simulink model "PCH_660_400_x3_6arm"  (R2018b)
settings: Solver=ode23t  StartTime=0.0  StopTime=0.1  RelTol=1e-3
undefined symbols (not defined in the file): fn, L_load, Lk, R12pu, R_load, Rmpu, Stv, U1, U2, X12pu, Xmpu
libraries: powerlib x65, powerlib_meascontrol x20, peRmsMeasurement x4
settings Model: Creator=K2  LastModifiedBy=sr1

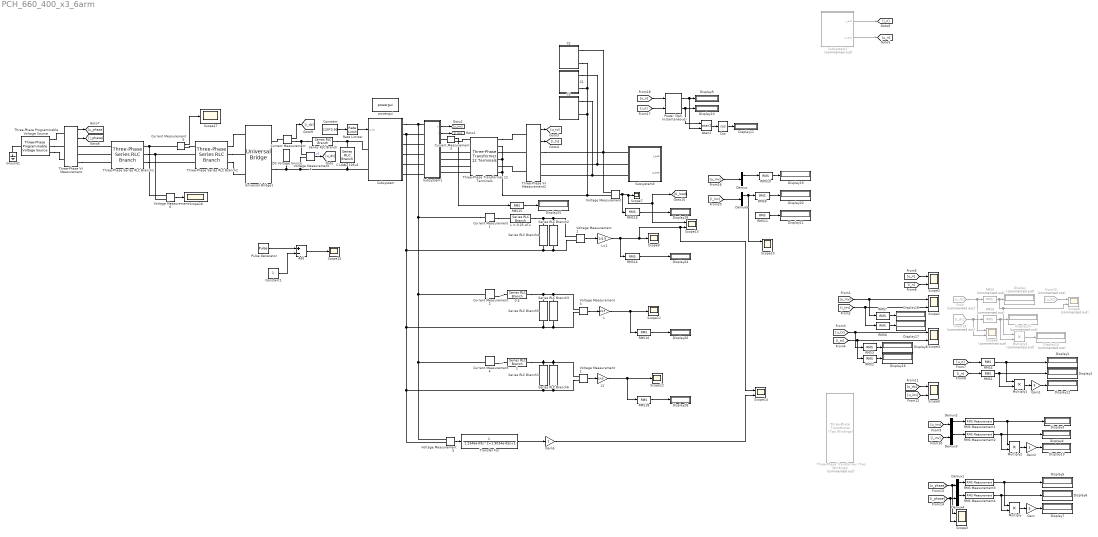
== system PCH_660_400_x3_6arm ==
  0.5 : powerlib/Elements/Series RLC Branch  LConnTagsString=__new0  RConnTagsString=__new0  BranchType=L  Resistance=0.0001  Inductance=Lk*2  SetiL0=off  InitialCurrent=0  Capacitance=1e-6  Setx0=off  InitialVoltage=0  Measurements=None
  1 : powerlib/Elements/Series RLC Branch  LConnTagsString=__new0  RConnTagsString=__new0  BranchType=L  Resistance=0.0001  Inductance=Lk*4  SetiL0=off  InitialCurrent=0  Capacitance=1e-6  Setx0=off  InitialVoltage=0  Measurements=None
  Add : Sum  Inputs=+-
  Atan2 : Trigonometry  Operator=atan2
  C1 : Subsystem
  C2 : Subsystem
  C3 : Subsystem
  Constant : Constant  Value=120*0.90  SampleTime=1e-6
  Constant1 : Constant
  Cos : Trigonometry  Operator=cos
  Current Measurement{,1..5} (6 alike) : powerlib/Measurements/Current Measurement  PhasorSimulation=off  OutputType=Complex  PSBequivalent=0
  DC Voltage Source : powerlib/Electrical Sources/DC Voltage Source  Amplitude=510*0.9  Measurements=None
  Demux{,1..5} (6 alike) : Demux  Outputs=3
  Display : Display  Commented=on
  Display{1..13,16..21,24..26,28..29} (24 alike) : Display
  Display14 : Display  Commented=on
  Display15 : Display  Commented=on
  From : From  Commented=on  GotoTag=u_dc
  From15 : From  Commented=on  GotoTag=u_dc
  From19 : From  Commented=on  GotoTag=i_dc
  Gain : Gain  Gain=3
  Gain1 : Gain  Gain=3
  Gain2 : Gain  Gain=3
  Gain5 : Gain
  Ground1 : powerlib/Elements/Ground  LConnTagsString=a
  L : Gain  Gain=1/4.5
  L = 0.25 мГн : powerlib/Elements/Series RLC Branch  LConnTagsString=__new0  RConnTagsString=__new0  BranchType=L  Resistance=0.002  Inductance=Lk  SetiL0=off  InitialCurrent=0  Capacitance=1e-6  Setx0=off  InitialVoltage=0  Measurements=None
  L1 : Gain  Gain=1/4.5
  "L=1 " : Gain  Gain=1/4.5
  Multiply : Product
  Multiply1 : Product
  Multiply2 : Product
  Multiply3 : Product  Commented=on
  "Power (3ph, Instantaneous)" : powerlib_meascontrol/Measurements/Power (3ph, Instantaneous)
      settings: SourceProductName=Simscape Power Systems
  Pulse Generator : DiscretePulseGenerator  PulseType=Time based  Amplitude=2  Period=1/400  PulseWidth=50
  RMS Measurement1 : peRmsMeasurement/RMS Measurement  LabelModeActiveChoice=Harmonic  F=400  SpecifyHarmonics=on  K=[1]  Ts=0
  RMS Measurement2 : peRmsMeasurement/RMS Measurement  LabelModeActiveChoice=Harmonic  F=400  SpecifyHarmonics=on  K=[1]  Ts=0
  RMS Measurement3 : peRmsMeasurement/RMS Measurement  LabelModeActiveChoice=Harmonic  F=50  SpecifyHarmonics=on  K=[1]  Ts=0
  RMS Measurement4 : peRmsMeasurement/RMS Measurement  LabelModeActiveChoice=Harmonic  F=50  SpecifyHarmonics=on  K=[1]  Ts=0
  RMS{1..4,6..7,9..11,14..16,18..19} (14 alike) : powerlib_meascontrol/Measurements/RMS  TrueRMS=on  Freq=400  RMSInit=0  Ts=0
  RMS5 : powerlib_meascontrol/Measurements/RMS  Commented=on  TrueRMS=on  Freq=300  RMSInit=0  Ts=0
  RMS8 : powerlib_meascontrol/Measurements/RMS  Commented=on  TrueRMS=on  Freq=300  RMSInit=0  Ts=0
  Rate Limiter : RateLimiter  RisingSlewLimit=50000  FallingSlewLimit=-50000  SampleTimeMode=inherited
  Scope{1..5,10,13..14} (8 alike) : Scope  NumInputPorts=2
  Scope{7,9,11..12,15..17} (7 alike) : Scope
  Scope6 : Scope  Commented=on  NumInputPorts=2
  Scope8 : Scope  Commented=on  NumInputPorts=2
  Series RLC Branch : powerlib/Elements/Series RLC Branch  LConnTagsString=__new0  RConnTagsString=__new0  BranchType=R  Resistance=0.0001  Inductance=250e-6  SetiL0=off  InitialCurrent=0  Capacitance=1e-6  Setx0=off  InitialVoltage=0  Measurements=None
  Series RLC Branch1 : powerlib/Elements/Series RLC Branch  LConnTagsString=__new0  RConnTagsString=__new0  BranchType=C  Resistance=0.0001  Inductance=250e-6  SetiL0=off  InitialCurrent=0  Capacitance=100e-6 / ((4.5)^2)  Setx0=off  InitialVoltage=0  Measurements=None
  Series RLC Branch2 : powerlib/Elements/Series RLC Branch  LConnTagsString=__new0  RConnTagsString=__new0  BranchType=R  Resistance=R_load * ((4.5)^2)  Inductance=250e-6  SetiL0=off  InitialCurrent=0  Capacitance=100e-6 / ((4.5)^2)  Setx0=off  InitialVoltage=0  Measurements=None
  Series RLC Branch3 : powerlib/Elements/Series RLC Branch  LConnTagsString=__new0  RConnTagsString=__new0  BranchType=R  Resistance=R_load * ((4.5)^2)  Inductance=250e-6  SetiL0=off  InitialCurrent=0  Capacitance=100e-6 / ((4.5)^2)  Setx0=off  InitialVoltage=0  Measurements=None
  Series RLC Branch4 : powerlib/Elements/Series RLC Branch  LConnTagsString=__new0  RConnTagsString=__new0  BranchType=C  Resistance=0.0001  Inductance=250e-6  SetiL0=off  InitialCurrent=0  Capacitance=100e-6 / ((4.5)^2)  Setx0=off  InitialVoltage=0  Measurements=None
  Series RLC Branch5 : powerlib/Elements/Series RLC Branch  LConnTagsString=__new0  RConnTagsString=__new0  BranchType=C  Resistance=0.0001  Inductance=250e-6  SetiL0=off  InitialCurrent=0  Capacitance=100e-6 / ((4.5)^2)  Setx0=off  InitialVoltage=0  Measurements=None
  Series RLC Branch6 : powerlib/Elements/Series RLC Branch  LConnTagsString=__new0  RConnTagsString=__new0  BranchType=R  Resistance=R_load * ((4.5)^2)  Inductance=250e-6  SetiL0=off  InitialCurrent=0  Capacitance=100e-6 / ((4.5)^2)  Setx0=off  InitialVoltage=0  Measurements=None
  Subsystem : Subsystem
  Subsystem1 : Subsystem
  Subsystem2 : Subsystem  Commented=on
  Subsystem3 : Subsystem
  Three-Phase Programmable Voltage Source : powerlib/Electrical Sources/Three-Phase Programmable Voltage Source  PositiveSequence=[660 0 50]  VariationEntity=None  VariationType=Table of time-amplitude pairs  VariationTypeAlt=Step  VariationStep=0.5  VariationRate=10  VariationMagnitude=0.3  VariationFrequency=2  VariationTiming=[1 2]  VariationPhaseA=off  Amplitudes=[1 0.8 1.2 1.0]  TimeValues=[0 0.1 0.15 0.2]  HarmonicGeneration=off  HarmonicA=[3 0.2 -25 0]  HarmonicB=[2 0.15 35 2]  Timing="[0.05  3]"  BusType=swing  Pref=0  Qref=0  Qmin=-inf  Qmax=inf
  Three-Phase Series RLC Branch1 : powerlib/Elements/Three-Phase Series RLC Branch  LConnTagsString=A|B|C  RConnTagsString=A|B|C  BranchType=R  Resistance=0.18  Inductance=150e-6  Capacitance=1e-6  Measurements=None
  Three-Phase Series RLC Branch2 : powerlib/Elements/Three-Phase Series RLC Branch  LConnTagsString=A|B|C  RConnTagsString=A|B|C  BranchType=L  Resistance=1  Inductance=150e-6  Capacitance=1e-6  Measurements=None
  Three-Phase Transformer (Two Windings) : powerlib/Elements/Three-Phase Transformer (Two Windings)  Commented=on  Winding1Connection=Yg  Winding2Connection=Yg  CoreType=Three single-phase transformers  SetSaturation=off  Hysteresis=off  DataFile='hysteresis'  SetInitialFlux=off  Measurements=None  UNITS=pu  NominalPower=[ 160e3 , 400 ]  Winding1=[690 , 0.002 , 0.08 ]  Winding2=[ 230 , 0.002 , 0.08 ]  Rm=500  Lm=500  L0=0.5  Saturation=[ 0,0 ; 0.0024,1.2 ; 1.0,1.52 ]  InitialFluxes=[ 0.8 , -0.8 , 0.7 ]  MoreParameters=off  BreakLoop=off  DataType=off  TransfoNumber=1
  Three-Phase V-I Measurement : powerlib/Measurements/Three-Phase V-I Measurement  VoltageMeasurement=phase-to-ground  SetLabelV=off  LabelV=Vabc  Vpu=off  VpuLL=off  CurrentMeasurement=yes  SetLabelI=off  LabelI=Iabc  Ipu=off  Pbase=100e6  Vbase=500e3  OutputType=Complex  PhasorSimulation=off  PSBequivalent=0
  Three-Phase V-I Measurement2 : powerlib/Measurements/Three-Phase V-I Measurement  VoltageMeasurement=phase-to-phase  SetLabelV=off  LabelV=Vabc  Vpu=off  VpuLL=off  CurrentMeasurement=yes  SetLabelI=off  LabelI=Iabc  Ipu=off  Pbase=100e6  Vbase=500e3  OutputType=Complex  PhasorSimulation=off  PSBequivalent=0
  Three-Phase Transformer 12 Terminals : powerlib/Elements/Three-Phase Transformer 12 Terminals  RatedPower=[ Stv fn ]  Winding1="[ U1 R12pu  X12pu ]"  Winding2=[ U2 R12pu X12pu]  RmXm=[ Rmpu Xmpu ]
      settings: SourceProductName=Simscape Power Systems  SourceProductBaseCode=PS
  Transfer Fcn : TransferFcn  Denominator=[1.2346e-09 1.9034e-05 1]
  Universal Bridge1 : powerlib/Power Electronics/Universal Bridge  Arms=3  SnubberResistance=1e5  SnubberCapacitance=inf  Device=Diodes  Ron=1e-3  Lon=0  ForwardVoltages="[  0  0  ]"  ForwardVoltage=0  GTOparameters=[ 10e-6 , 20e-6 ]  IGBTparameters=[ 1e-6 , 2e-6 ]  Measurements=None  Measurements_2=None  converterType=Rectifier
  Voltage Measurement{,1..6} (7 alike) : powerlib/Measurements/Voltage Measurement  PhasorSimulation=off  OutputType=Complex  PSBequivalent=0
  powergui : powerlib/powergui  Priority=1  SimulationMode=Discrete  SampleTime=1e-6  frequency=60  Iterations=50  frequencyindice=0  Pbase=100e6  ErrMax=1e-4  UnitsV=kV  UnitsW=MW  buscounter=0  FunctionMessages=off  echomessages=off  EnableUseOfTLC=off  CurrentSourceSwitches=off  DisableSnubberDevices=off  DisableRonSwitches=off  DisableVfSwitches=off  DisplayEquations=off  SolverType=Tustin/Backward Euler (TBE)  Interpol=off  ExternalGateDelay=off  methode=off  Ts=100  x0status=blocks  SPID=on  SwTol=0  HookPort=off  RestoreLinks=warning  ResistiveCurrentMeasurement=off  Frange=[0:2:500]  Ylog=off  Xlog=on  ShowGrid=off  save=off  variable=ZData  structure=logsout  ZoomFFT=off  StartTime=0.08  cycles=4  DisplayStyle=1  fundamental=400  FreqAxis=off  MaxFrequency=4000  frequencyindicesteady=1  RmsSteady=1  display=off
  С LOAD 105u1 : powerlib/Elements/Series RLC Branch  LConnTagsString=__new0  RConnTagsString=__new0  BranchType=C  Resistance=250*250/50e3  Inductance=1e-3  SetiL0=off  InitialCurrent=0  Capacitance=11400e-6  Setx0=on  InitialVoltage=800  Measurements=None
  wires:
  Three-Phase V-I Measurement/1 -> [u_phase]
  Three-Phase V-I Measurement/2 -> [i_phase]
  Voltage Measurement4/1 -> [u_dc]  "u1"
  Three-Phase V-I Measurement2/1 -> [u_tv]
  Three-Phase V-I Measurement2/2 -> [i_tv]
  Constant/1 -> Rate Limiter/1
  [u_n] -> Scope2/1
  [i_n] -> Scope2/2
  [u_inv] -> RMS7/1, Scope1/1
  [i_inv] -> RMS6/1, Scope1/2
  [u_tv] -> Scope4/1, RMS3/1
  [i_tv] -> Scope4/2, RMS2/1
  [u_n] -> RMS4/1
  [i_n] -> RMS1/1
  [i_inv] -> Demux3/1
  [u_inv] -> Demux2/1
  [u_dc] -> Scope5/1
  [u_inv] -> Scope5/2
  Rate Limiter/1 -> Subsystem/1(u in)
  RMS5/1 -> Multiply3/1, Scope6/2, Display/1
  RMS Measurement3/1 -> Multiply/1, Display5/1
  RMS Measurement4/1 -> Multiply/2, Display6/1
  Multiply/1 -> Gain/1
  Gain/1 -> Display7/1
  From15/1 -> Scope6/1
  Subsystem1/2(i) -> [i_inv]
  Subsystem1/1(v) -> [u_inv]
  Cos/1 -> Display11/1
  "Power (3ph, Instantaneous)"/2 -> Atan2/1, Display10/1
  Atan2/1 -> Cos/1
  "Power (3ph, Instantaneous)"/1 -> Atan2/2, Display9/1
  [i_n] -> "Power (3ph, Instantaneous)"/2
  [u_n] -> "Power (3ph, Instantaneous)"/1
  Gain1/1 -> Display12/1
  RMS1/1 -> Display2/1, Multiply1/2
  RMS4/1 -> Display1/1, Multiply1/1
  Multiply1/1 -> Gain1/1
  Gain2/1 -> Display13/1
  RMS Measurement2/1 -> Multiply2/2, Display4/1
  RMS Measurement1/1 -> Multiply2/1, Display3/1
  Multiply2/1 -> Gain2/1
  Current Measurement/1 -> [i_dc]
  RMS8/1 -> Multiply3/2, Display14/1
  Multiply3/1 -> Display15/1
  From/1 -> Scope8/1, RMS5/1
  From19/1 -> Scope8/2, RMS8/1
  Demux2/1 -> RMS Measurement1/1
  Demux3/1 -> RMS Measurement2/1
  Demux4/1 -> RMS Measurement4/1
  Demux1/1 -> RMS Measurement3/1
  [u_phase] -> Scope3/1, Demux1/1
  [i_phase] -> Scope3/2, Demux4/1
  RMS3/1 -> Display8/1
  RMS2/1 -> Display16/1
  RMS6/1 -> Display17/1
  RMS7/1 -> Display18/1
  Voltage Measurement1/1 -> "L=1 "/1
  Voltage Measurement3/1 -> L/1
  Voltage Measurement5/1 -> Transfer Fcn/1
  Transfer Fcn/1 -> Gain5/1
  "L=1 "/1 -> RMS14/1, Scope14/1, Scope13/2, Scope9/1
  RMS10/1 -> Display19/1
  [u_inv] -> Demux/1
  Demux/1 -> RMS10/1
  RMS9/1 -> Display20/1
  RMS11/1 -> Display21/1
  Demux5/1 -> Scope10/1, RMS9/1
  [i_inv] -> Demux5/1
  Subsystem2/1(i_out) -> [i_n]
  Subsystem2/2(u_out) -> [u_n]
  RMS14/1 -> Display24/1
  RMS16/1 -> Display26/1
  RMS15/1 -> Display25/1
  Current Measurement3/1 -> RMS15/1
  Voltage Measurement2/1 -> L1/1
  L1/1 -> RMS18/1, Scope12/1
  RMS18/1 -> Display28/1
  RMS19/1 -> Display29/1
  Voltage Measurement/1 -> [U_load], Scope13/1, Scope7/1, RMS19/1
  Gain5/1 -> Scope14/2
  L/1 -> RMS16/1, Scope11/1
  Pulse Generator/1 -> Add/1
  Constant1/1 -> Add/2
  Add/1 -> Scope15/1
  Voltage Measurement6/1 -> Scope16/1
  Current Measurement5/1 -> Scope17/1
  connections:
  Three-Phase Programmable Voltage Source/RConn3 -- Three-Phase V-I Measurement/LConn3
  Three-Phase Programmable Voltage Source/RConn2 -- Three-Phase V-I Measurement/LConn2
  Three-Phase Series RLC Branch2/RConn3 -- Universal Bridge1/LConn3
  Three-Phase Programmable Voltage Source/LConn1 -- Ground1/LConn1
  Three-Phase Series RLC Branch2/RConn1 -- Universal Bridge1/LConn1
  Three-Phase Programmable Voltage Source/RConn1 -- Three-Phase V-I Measurement/LConn1
  Three-Phase Series RLC Branch2/RConn2 -- Universal Bridge1/LConn2
  Series RLC Branch/LConn1 -- Current Measurement/RConn1 -- Voltage Measurement4/LConn1
  Universal Bridge1/RConn2 -- Subsystem/LConn2 -- С LOAD 105u1/RConn1 -- Voltage Measurement4/LConn2 -- DC Voltage Source/LConn1
  Three-Phase V-I Measurement2/RConn1 -- Subsystem3/LConn1 -- Voltage Measurement/LConn1 -- C2/LConn1
  C3/LConn1 -- Three-Phase V-I Measurement2/RConn3 -- Subsystem3/LConn3
  Three-Phase V-I Measurement2/LConn2 -- Three-Phase Transformer 12 Terminals/RConn3
  Three-Phase Transformer 12 Terminals/RConn1 -- Three-Phase V-I Measurement2/LConn1
  Series RLC Branch/RConn1 -- Subsystem/LConn1 -- С LOAD 105u1/LConn1
  Voltage Measurement2/LConn2 -- Series RLC Branch5/RConn1 -- Series RLC Branch3/RConn1 -- Voltage Measurement3/LConn2 -- Series RLC Branch2/RConn1 -- Voltage Measurement1/LConn2 -- Series RLC Branch4/RConn1 -- Subsystem/RConn2 -- Subsystem1/LConn2 -- Voltage Measurement5/LConn2 -- Series RLC Branch1/RConn1 -- Series RLC Branch6/RConn1
  Three-Phase Transformer 12 Terminals/LConn4 -- Subsystem1/RConn4
  Three-Phase Transformer 12 Terminals/LConn5 -- Subsystem1/RConn5
  Three-Phase Transformer 12 Terminals/LConn3 -- Subsystem1/RConn3
  Current Measurement1/LConn1 -- Voltage Measurement5/LConn1 -- Current Measurement4/LConn1 -- Current Measurement2/LConn1 -- Subsystem/RConn1 -- Subsystem1/LConn1
  Subsystem1/LConn3 -- Subsystem/RConn3
  Subsystem1/LConn4 -- Subsystem/RConn4
  Subsystem1/LConn5 -- Subsystem/RConn5
  Subsystem1/LConn6 -- Subsystem/RConn6
  Current Measurement/LConn1 -- Universal Bridge1/RConn1
  Three-Phase V-I Measurement2/LConn3 -- Three-Phase Transformer 12 Terminals/RConn5
  C1/LConn1 -- Three-Phase V-I Measurement2/RConn2 -- Subsystem3/LConn2
  C2/LConn3 -- C1/LConn3 -- C3/LConn3 -- Voltage Measurement/LConn2 -- Three-Phase Transformer 12 Terminals/RConn2 -- Three-Phase Transformer 12 Terminals/RConn4 -- Three-Phase Transformer 12 Terminals/RConn6
  L = 0.25 мГн/RConn1 -- Series RLC Branch2/LConn1 -- Voltage Measurement1/LConn1 -- Series RLC Branch4/LConn1
  Current Measurement1/RConn1 -- L = 0.25 мГн/LConn1
  Three-Phase Transformer 12 Terminals/LConn2 -- Subsystem1/RConn2
  Three-Phase Transformer 12 Terminals/LConn6 -- Subsystem1/RConn6
  Current Measurement2/RConn1 -- 0.5/LConn1
  Current Measurement3/RConn1 -- Three-Phase Transformer 12 Terminals/LConn1
  Current Measurement3/LConn1 -- Subsystem1/RConn1
  Series RLC Branch1/LConn1 -- Series RLC Branch6/LConn1 -- Voltage Measurement2/LConn1 -- 1/RConn1
  Current Measurement4/RConn1 -- 1/LConn1
  0.5/RConn1 -- Series RLC Branch3/LConn1 -- Voltage Measurement3/LConn1 -- Series RLC Branch5/LConn1
  Three-Phase Series RLC Branch1/RConn1 -- Current Measurement5/LConn1 -- Voltage Measurement6/LConn1
  Three-Phase Series RLC Branch1/LConn1 -- Three-Phase V-I Measurement/RConn1
  Three-Phase Series RLC Branch1/RConn2 -- Three-Phase Series RLC Branch2/LConn2 -- Voltage Measurement6/LConn2
  Three-Phase Series RLC Branch1/LConn2 -- Three-Phase V-I Measurement/RConn2
  Three-Phase V-I Measurement/RConn3 -- Three-Phase Series RLC Branch1/LConn3
  Three-Phase Series RLC Branch1/RConn3 -- Three-Phase Series RLC Branch2/LConn3
  Current Measurement5/RConn1 -- Three-Phase Series RLC Branch2/LConn1

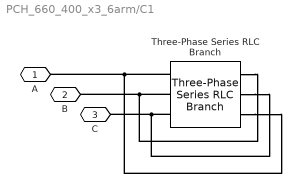
== system PCH_660_400_x3_6arm/C1 ==
  Three-Phase Series RLC Branch : powerlib/Elements/Three-Phase Series RLC Branch  LConnTagsString=A|B|C  RConnTagsString=A|B|C  BranchType=C  Resistance=0.001  Inductance=100e-6  Capacitance=100e-6  Measurements=None
  A : PMIOPort  Side=Left
  B : PMIOPort  Port=2  Side=Left
  C : PMIOPort  Port=3  Side=Left
  connections:
  Three-Phase Series RLC Branch/LConn3 -- Three-Phase Series RLC Branch/RConn2 -- C/RConn1
  Three-Phase Series RLC Branch/LConn1 -- Three-Phase Series RLC Branch/RConn3 -- A/RConn1
  Three-Phase Series RLC Branch/LConn2 -- Three-Phase Series RLC Branch/RConn1 -- B/RConn1

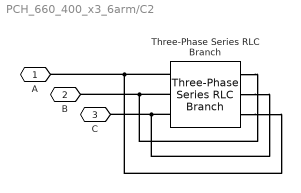
== system PCH_660_400_x3_6arm/C2 ==
  Three-Phase Series RLC Branch : powerlib/Elements/Three-Phase Series RLC Branch  LConnTagsString=A|B|C  RConnTagsString=A|B|C  BranchType=C  Resistance=0.001  Inductance=100e-6  Capacitance=100e-6  Measurements=None
  A : PMIOPort  Side=Left
  B : PMIOPort  Port=2  Side=Left
  C : PMIOPort  Port=3  Side=Left
  connections:
  Three-Phase Series RLC Branch/LConn3 -- Three-Phase Series RLC Branch/RConn2 -- C/RConn1
  Three-Phase Series RLC Branch/LConn1 -- Three-Phase Series RLC Branch/RConn3 -- A/RConn1
  Three-Phase Series RLC Branch/LConn2 -- Three-Phase Series RLC Branch/RConn1 -- B/RConn1

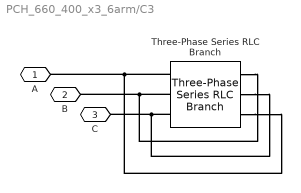
== system PCH_660_400_x3_6arm/C3 ==
  Three-Phase Series RLC Branch : powerlib/Elements/Three-Phase Series RLC Branch  LConnTagsString=A|B|C  RConnTagsString=A|B|C  BranchType=C  Resistance=0.001  Inductance=100e-6  Capacitance=100e-6  Measurements=None
  A : PMIOPort  Side=Left
  B : PMIOPort  Port=2  Side=Left
  C : PMIOPort  Port=3  Side=Left
  connections:
  Three-Phase Series RLC Branch/LConn3 -- Three-Phase Series RLC Branch/RConn2 -- C/RConn1
  Three-Phase Series RLC Branch/LConn1 -- Three-Phase Series RLC Branch/RConn3 -- A/RConn1
  Three-Phase Series RLC Branch/LConn2 -- Three-Phase Series RLC Branch/RConn1 -- B/RConn1

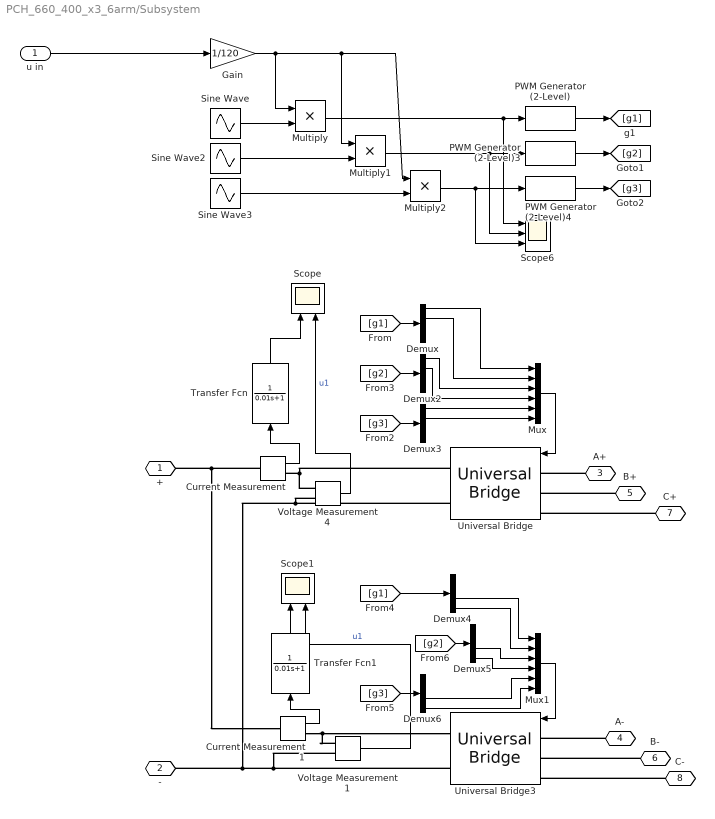
== system PCH_660_400_x3_6arm/Subsystem ==
  u in : Inport
  Current Measurement : powerlib/Measurements/Current Measurement  PhasorSimulation=off  OutputType=Complex  PSBequivalent=0
  Current Measurement1 : powerlib/Measurements/Current Measurement  PhasorSimulation=off  OutputType=Complex  PSBequivalent=0
  Demux{,2..6} (6 alike) : Demux
  Gain : Gain  Gain=1/120
  Multiply : Product
  Multiply1 : Product
  Multiply2 : Product
  Mux : Mux  Inputs=6
  Mux1 : Mux  Inputs=6
  PWM Generator (2-Level) : powerlib_meascontrol/Pulse & Signal Generators/PWM Generator (2-Level)  ModulatorType=Single-phase full-bridge (4 pulses)  ModulatorMode=Unsynchronized  Fc=5600  Pc=0  nF=27  MinMax="[ -1  1 ]"  SamplingTechnique=Natural  ModulatingSignals=off  m=0.8  Freq=60  Phase=0  Ts=0  ShowCarrierOutport=off
      settings: SourceProductName=Simscape Power Systems
  PWM Generator (2-Level)3 : powerlib_meascontrol/Pulse & Signal Generators/PWM Generator (2-Level)  ModulatorType=Single-phase full-bridge (4 pulses)  ModulatorMode=Unsynchronized  Fc=5600  Pc=120  nF=27  MinMax="[ -1  1 ]"  SamplingTechnique=Natural  ModulatingSignals=off  m=0.8  Freq=60  Phase=0  Ts=0  ShowCarrierOutport=off
      settings: SourceProductName=Simscape Power Systems
  PWM Generator (2-Level)4 : powerlib_meascontrol/Pulse & Signal Generators/PWM Generator (2-Level)  ModulatorType=Single-phase full-bridge (4 pulses)  ModulatorMode=Unsynchronized  Fc=5600  Pc=-120  nF=27  MinMax="[ -1  1 ]"  SamplingTechnique=Natural  ModulatingSignals=off  m=0.8  Freq=60  Phase=0  Ts=0  ShowCarrierOutport=off
      settings: SourceProductName=Simscape Power Systems
  Scope : Scope  NumInputPorts=2
  Scope1 : Scope  NumInputPorts=2
  Scope6 : Scope  NumInputPorts=3
  Sine Wave : Sin  Frequency=400*2*pi  SampleTime=0
  Sine Wave2 : Sin  Frequency=400*2*pi  Phase=-2*pi/3  SampleTime=0
  Sine Wave3 : Sin  Frequency=400*2*pi  Phase=2*pi/3  SampleTime=0
  Transfer Fcn : TransferFcn  Denominator=[0.01 1]
  Transfer Fcn1 : TransferFcn  Denominator=[0.01 1]
  Universal Bridge : powerlib/Power Electronics/Universal Bridge  Arms=3  SnubberResistance=1e5  SnubberCapacitance=inf  Device=IGBT / Diodes  Ron=5e-3  Lon=0  ForwardVoltages="[  1.5  1  ]"  ForwardVoltage=0  GTOparameters=[ 10e-6 , 20e-6 ]  IGBTparameters=[ 1e-6 , 2e-6 ]  Measurements=Device currents  Measurements_2=None  converterType=Rectifier
  Universal Bridge3 : powerlib/Power Electronics/Universal Bridge  Arms=3  SnubberResistance=1e5  SnubberCapacitance=inf  Device=IGBT / Diodes  Ron=5e-3  Lon=0  ForwardVoltages="[  1.5  1  ]"  ForwardVoltage=0  GTOparameters=[ 10e-6 , 20e-6 ]  IGBTparameters=[ 1e-6 , 2e-6 ]  Measurements=Device currents  Measurements_2=None  converterType=Rectifier
  Voltage Measurement1 : powerlib/Measurements/Voltage Measurement  PhasorSimulation=off  OutputType=Complex  PSBequivalent=0
  Voltage Measurement4 : powerlib/Measurements/Voltage Measurement  PhasorSimulation=off  OutputType=Complex  PSBequivalent=0
  + : PMIOPort  Side=Left
  - : PMIOPort  Port=2  Side=Left
  A+ : PMIOPort  Port=3  Side=Right
  A- : PMIOPort  Port=4  Side=Right
  B+ : PMIOPort  Port=5  Side=Right
  B- : PMIOPort  Port=6  Side=Right
  C+ : PMIOPort  Port=7  Side=Right
  C- : PMIOPort  Port=8  Side=Right
  wires:
  Mux1/1 -> Universal Bridge3/1
  Mux/1 -> Universal Bridge/1
  PWM Generator (2-Level)/1 -> [g1]
  Gain/1 -> Multiply2/1, Multiply1/1, Multiply/1
  u in/1 -> Gain/1
  Multiply/1 -> Scope6/1, PWM Generator (2-Level)/1
  Sine Wave/1 -> Multiply/2
  Sine Wave2/1 -> Multiply1/2
  Sine Wave3/1 -> Multiply2/2
  Multiply2/1 -> Scope6/3, PWM Generator (2-Level)4/1
  Multiply1/1 -> Scope6/2, PWM Generator (2-Level)3/1
  PWM Generator (2-Level)4/1 -> [g3]
  PWM Generator (2-Level)3/1 -> [g2]
  [g1] -> Demux/1
  Demux/1 -> Mux/1
  Demux/2 -> Mux/2
  [g2] -> Demux2/1
  Demux2/1 -> Mux/3
  Demux2/2 -> Mux/4
  [g3] -> Demux3/1
  Demux3/2 -> Mux/6
  Demux3/1 -> Mux/5
  [g1] -> Demux4/1
  Demux4/3 -> Mux1/1
  [g3] -> Demux6/1
  Demux5/4 -> Mux1/4
  Demux4/4 -> Mux1/2
  Demux5/3 -> Mux1/3
  Demux6/4 -> Mux1/6
  [g2] -> Demux5/1
  Demux6/3 -> Mux1/5
  Current Measurement/1 -> Transfer Fcn/1
  Voltage Measurement4/1 -> Scope/2  "u1"
  Voltage Measurement1/1 -> Scope1/2  "u1"
  Current Measurement1/1 -> Transfer Fcn1/1
  Transfer Fcn/1 -> Scope/1
  Transfer Fcn1/1 -> Scope1/1
  connections:
  +/RConn1 -- Current Measurement1/LConn1 -- Current Measurement/LConn1
  A+/RConn1 -- Universal Bridge/LConn1
  Universal Bridge/RConn2 -- Voltage Measurement4/LConn2 -- Universal Bridge3/RConn2 -- Voltage Measurement1/LConn2 -- -/RConn1
  B+/RConn1 -- Universal Bridge/LConn2
  C+/RConn1 -- Universal Bridge/LConn3
  C-/RConn1 -- Universal Bridge3/LConn3
  B-/RConn1 -- Universal Bridge3/LConn2
  A-/RConn1 -- Universal Bridge3/LConn1
  Voltage Measurement4/LConn1 -- Universal Bridge/RConn1 -- Current Measurement/RConn1
  Current Measurement1/RConn1 -- Universal Bridge3/RConn1 -- Voltage Measurement1/LConn1

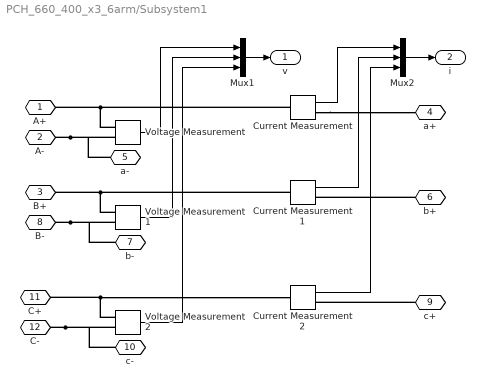
== system PCH_660_400_x3_6arm/Subsystem1 ==
  Current Measurement : powerlib/Measurements/Current Measurement  PhasorSimulation=off  OutputType=Complex  PSBequivalent=0
  Current Measurement1 : powerlib/Measurements/Current Measurement  PhasorSimulation=off  OutputType=Complex  PSBequivalent=0
  Current Measurement2 : powerlib/Measurements/Current Measurement  PhasorSimulation=off  OutputType=Complex  PSBequivalent=0
  Mux1 : Mux  Inputs=3
  Mux2 : Mux  Inputs=3
  Voltage Measurement : powerlib/Measurements/Voltage Measurement  PhasorSimulation=off  OutputType=Complex  PSBequivalent=0
  Voltage Measurement1 : powerlib/Measurements/Voltage Measurement  PhasorSimulation=off  OutputType=Complex  PSBequivalent=0
  Voltage Measurement2 : powerlib/Measurements/Voltage Measurement  PhasorSimulation=off  OutputType=Complex  PSBequivalent=0
  A+ : PMIOPort  Side=Left
  A- : PMIOPort  Port=2  Side=Left
  B+ : PMIOPort  Port=3  Side=Left
  a+ : PMIOPort  Port=4  Side=Right
  a- : PMIOPort  Port=5  Side=Right
  b+ : PMIOPort  Port=6  Side=Right
  b- : PMIOPort  Port=7  Side=Right
  B- : PMIOPort  Port=8  Side=Left
  c+ : PMIOPort  Port=9  Side=Right
  c- : PMIOPort  Port=10  Side=Right
  C+ : PMIOPort  Port=11  Side=Left
  C- : PMIOPort  Port=12  Side=Left
  v : Outport
  i : Outport  Port=2
  wires:
  Voltage Measurement1/1 -> Mux1/2
  Current Measurement2/1 -> Mux2/3
  Voltage Measurement2/1 -> Mux1/3
  Current Measurement/1 -> Mux2/1
  Voltage Measurement/1 -> Mux1/1
  Mux1/1 -> v/1
  Current Measurement1/1 -> Mux2/2
  Mux2/1 -> i/1
  connections:
  Current Measurement/RConn1 -- a+/RConn1
  Current Measurement/LConn1 -- Voltage Measurement/LConn1 -- A+/RConn1
  Voltage Measurement2/LConn1 -- Current Measurement2/LConn1 -- C+/RConn1
  c+/RConn1 -- Current Measurement2/RConn1
  Current Measurement1/LConn1 -- Voltage Measurement1/LConn1 -- B+/RConn1
  B-/RConn1 -- Voltage Measurement1/LConn2 -- b-/RConn1
  b+/RConn1 -- Current Measurement1/RConn1
  A-/RConn1 -- Voltage Measurement/LConn2 -- a-/RConn1
  C-/RConn1 -- Voltage Measurement2/LConn2 -- c-/RConn1

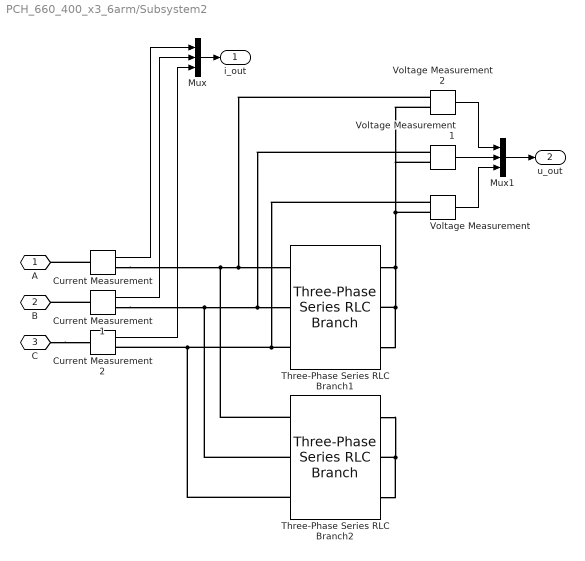
== system PCH_660_400_x3_6arm/Subsystem2 ==
  Current Measurement : powerlib/Measurements/Current Measurement  PhasorSimulation=off  OutputType=Complex  PSBequivalent=0
  Current Measurement1 : powerlib/Measurements/Current Measurement  PhasorSimulation=off  OutputType=Complex  PSBequivalent=0
  Current Measurement2 : powerlib/Measurements/Current Measurement  PhasorSimulation=off  OutputType=Complex  PSBequivalent=0
  Mux : Mux  Inputs=3
  Mux1 : Mux  Inputs=3
  Three-Phase Series RLC Branch1 : powerlib/Elements/Three-Phase Series RLC Branch  LConnTagsString=A|B|C  RConnTagsString=A|B|C  BranchType=RL  Resistance=R_load  Inductance=L_load  Capacitance=105e-6  Measurements=None
  Three-Phase Series RLC Branch2 : powerlib/Elements/Three-Phase Series RLC Branch  LConnTagsString=A|B|C  RConnTagsString=A|B|C  BranchType=R  Resistance=2.4  Inductance=L_load  Capacitance=105e-6  Measurements=None
  Voltage Measurement : powerlib/Measurements/Voltage Measurement  PhasorSimulation=off  OutputType=Complex  PSBequivalent=0
  Voltage Measurement1 : powerlib/Measurements/Voltage Measurement  PhasorSimulation=off  OutputType=Complex  PSBequivalent=0
  Voltage Measurement2 : powerlib/Measurements/Voltage Measurement  PhasorSimulation=off  OutputType=Complex  PSBequivalent=0
  A : PMIOPort  Side=Left
  B : PMIOPort  Port=2  Side=Left
  C : PMIOPort  Port=3  Side=Left
  i_out : Outport
  u_out : Outport  Port=2
  wires:
  Mux/1 -> i_out/1
  Current Measurement/1 -> Mux/1
  Current Measurement1/1 -> Mux/2
  Current Measurement2/1 -> Mux/3
  Voltage Measurement1/1 -> Mux1/2
  Voltage Measurement2/1 -> Mux1/1
  Voltage Measurement/1 -> Mux1/3
  Mux1/1 -> u_out/1
  connections:
  Three-Phase Series RLC Branch1/RConn3 -- Voltage Measurement2/LConn2 -- Voltage Measurement1/LConn2 -- Voltage Measurement/LConn2 -- Three-Phase Series RLC Branch1/RConn1 -- Three-Phase Series RLC Branch1/RConn2
  Current Measurement1/LConn1 -- B/RConn1
  Current Measurement/LConn1 -- A/RConn1
  Three-Phase Series RLC Branch1/LConn3 -- Voltage Measurement/LConn1 -- Three-Phase Series RLC Branch2/LConn3 -- Current Measurement2/RConn1
  Current Measurement/RConn1 -- Three-Phase Series RLC Branch2/LConn1 -- Voltage Measurement2/LConn1 -- Three-Phase Series RLC Branch1/LConn1
  Current Measurement1/RConn1 -- Three-Phase Series RLC Branch2/LConn2 -- Voltage Measurement1/LConn1 -- Three-Phase Series RLC Branch1/LConn2
  C/RConn1 -- Current Measurement2/LConn1
  Three-Phase Series RLC Branch2/RConn1 -- Three-Phase Series RLC Branch2/RConn3 -- Three-Phase Series RLC Branch2/RConn2

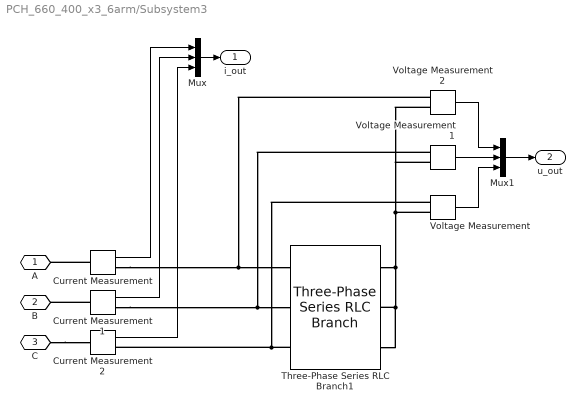
== system PCH_660_400_x3_6arm/Subsystem3 ==
  Current Measurement : powerlib/Measurements/Current Measurement  PhasorSimulation=off  OutputType=Complex  PSBequivalent=0
  Current Measurement1 : powerlib/Measurements/Current Measurement  PhasorSimulation=off  OutputType=Complex  PSBequivalent=0
  Current Measurement2 : powerlib/Measurements/Current Measurement  PhasorSimulation=off  OutputType=Complex  PSBequivalent=0
  Mux : Mux  Inputs=3
  Mux1 : Mux  Inputs=3
  Three-Phase Series RLC Branch1 : powerlib/Elements/Three-Phase Series RLC Branch  LConnTagsString=A|B|C  RConnTagsString=A|B|C  BranchType=R  Resistance=R_load  Inductance=L_load  Capacitance=105e-6  Measurements=None
  Voltage Measurement : powerlib/Measurements/Voltage Measurement  PhasorSimulation=off  OutputType=Complex  PSBequivalent=0
  Voltage Measurement1 : powerlib/Measurements/Voltage Measurement  PhasorSimulation=off  OutputType=Complex  PSBequivalent=0
  Voltage Measurement2 : powerlib/Measurements/Voltage Measurement  PhasorSimulation=off  OutputType=Complex  PSBequivalent=0
  A : PMIOPort  Side=Left
  B : PMIOPort  Port=2  Side=Left
  C : PMIOPort  Port=3  Side=Left
  i_out : Outport
  u_out : Outport  Port=2
  wires:
  Mux/1 -> i_out/1
  Current Measurement/1 -> Mux/1
  Current Measurement1/1 -> Mux/2
  Current Measurement2/1 -> Mux/3
  Voltage Measurement1/1 -> Mux1/2
  Voltage Measurement2/1 -> Mux1/1
  Voltage Measurement/1 -> Mux1/3
  Mux1/1 -> u_out/1
  connections:
  Three-Phase Series RLC Branch1/RConn3 -- Voltage Measurement2/LConn2 -- Voltage Measurement1/LConn2 -- Voltage Measurement/LConn2 -- Three-Phase Series RLC Branch1/RConn1 -- Three-Phase Series RLC Branch1/RConn2
  Current Measurement1/LConn1 -- B/RConn1
  Current Measurement/LConn1 -- A/RConn1
  Three-Phase Series RLC Branch1/LConn3 -- Voltage Measurement/LConn1 -- Current Measurement2/RConn1
  Current Measurement/RConn1 -- Voltage Measurement2/LConn1 -- Three-Phase Series RLC Branch1/LConn1
  Current Measurement1/RConn1 -- Voltage Measurement1/LConn1 -- Three-Phase Series RLC Branch1/LConn2
  C/RConn1 -- Current Measurement2/LConn1
